simulink model "doc_compander"  (R2014a)
settings: Solver=ode45  StartTime=0.0  StopTime=80  RelTol=1e-3
undefined symbols (not defined in the file or in its folder): sig
libraries: commsrccod2 x3, simulink x2, dspsrcs4 x1
settings Model: Creator=The MathWorks Inc.
settings DataIOCC: SignalLoggingSaveFormat=ModelDataLogs  SignalLoggingName=logsOut
settings OptimizationCC: BlockReduction=off  BooleanDataType=off  ExpressionDepthLimit=2147483647
settings DebuggingCC: SaveWithParameterizedLinksMsg=none  UnderspecifiedInitializationDetection=Classic  SignalResolutionControl=TryResolveAllWithWarning  SolverPrmCheckMsg=none  MultiTaskDSMMsg=warning  MultiTaskCondExecSysMsg=none  FcnCallInpInsideContextMsg=UseLocalSettings  StateNameClashWarn=warning  StrictBusMsg=None
settings HardwareCC: TargetUnknown=on
settings RTWCC: IncludeERTFirstTime=on
settings GRTTargetCC: TargetFcnLib=iso_c_tmw.mat  CombineOutputUpdateFcns=off  GRTInterface=on

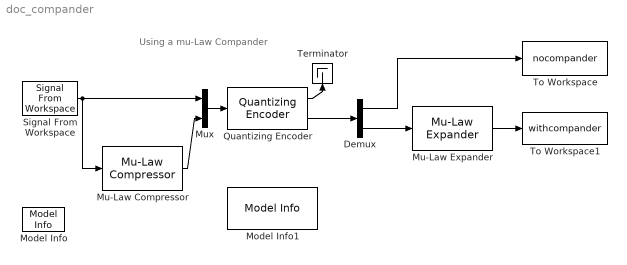
== system doc_compander ==
  note: Using a mu-Law Compander
  Demux : Demux  Outputs=2
  Model Info : simulink/Model-Wide Utilities/Model Info  InitialBlockCM=None  BlockCM=none  Frame=on  DisplayStringWithTags=Info  HorizontalTextAlignment=Center  LeftAlignmentValue=0.5  SourceBlockDiagram=doc_compander  TagMaxNumber=20
  Model Info1 : simulink/Model-Wide Utilities/Model Info  InitialBlockCM=None  BlockCM=none  Frame=on  DisplayStringWithTags=Info  HorizontalTextAlignment=Center  LeftAlignmentValue=0.5  SourceBlockDiagram=doc_compander  TagMaxNumber=20
  Mu-Law Compressor : commsrccod2/Mu-Law Compressor  mu=255  V=max(sig)
  Mu-Law Expander : commsrccod2/Mu-Law Expander  mu=255  V=ceil(max(sig))
  Mux : Mux  Inputs=2
  Quantizing Encoder : commsrccod2/Quantizing Encoder  partition=0:floor(max(sig))  codebook=0:ceil(max(sig))  idxDType=double
  Signal From Workspace : dspsrcs4/Signal From Workspace  X=sig  Ts=1  nsamps=1  OutputAfterFinalValue=Setting to zero  ignoreOrWarnInputAndFrameLengths=off
  Terminator : Terminator
  To Workspace : ToWorkspace  VariableName=nocompander  SampleTime=-1
  To Workspace1 : ToWorkspace  VariableName=withcompander  SampleTime=-1
  wires:
  Signal From Workspace/1 -> Mux/1, Mu-Law Compressor/1
  Mu-Law Compressor/1 -> Mux/2
  Mux/1 -> Quantizing Encoder/1
  Quantizing Encoder/1 -> Terminator/1
  Quantizing Encoder/2 -> Demux/1
  Demux/2 -> Mu-Law Expander/1
  Mu-Law Expander/1 -> To Workspace1/1
  Demux/1 -> To Workspace/1
